simulink model "intro_sim_d"  (R2021b)
settings: Solver=VariableStepAuto  StartTime=0.0  StopTime=10.0  RelTol=1e-3
settings Model: Creator=Juho  LastModifiedBy=Juho

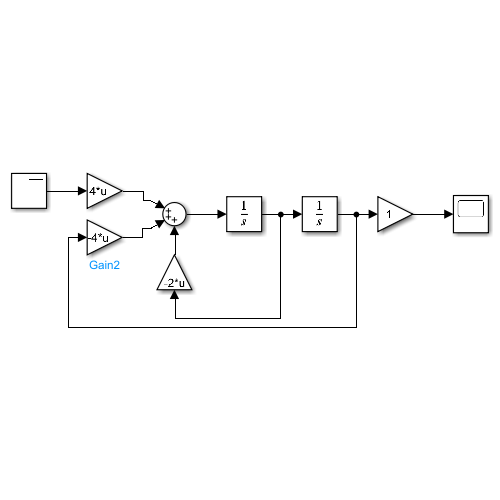
[thumbnail: Simulink's stored preview of the top-level diagram]
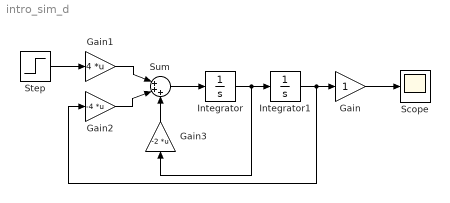
== system intro_sim_d ==
  Gain : Gain
  Gain1 : Gain  Gain=4  Multiplication=Matrix(K*u)
  Gain2 : Gain  Gain=-4  Multiplication=Matrix(K*u)
  Gain3 : Gain  Gain=-2  Multiplication=Matrix(K*u)
  Integrator : Integrator
  Integrator1 : Integrator
  Scope : Scope
  Step : Step  Time=0  SampleTime=0
  Sum : Sum  Inputs=|+++
  wires:
  Gain/1 -> Scope/1
  Sum/1 -> Integrator/1
  Integrator1/1 -> Gain2/1, Gain/1
  Integrator/1 -> Gain3/1, Integrator1/1
  Gain3/1 -> Sum/3
  Gain2/1 -> Sum/2
  Gain1/1 -> Sum/1
  Step/1 -> Gain1/1
